simulink model "onlympc"  (R2025a)
settings: Solver=FixedStepAuto  StartTime=0.0  StopTime=inf  FixedStep=0.01  RelTol=1e-3  EnableMultiTasking=on
InitFcn:
  | load2slx
model workspace (MAT data in the model file):
  F = [1.0101  0  0; 0  1.0101  0; 0  0  1.0101; 1.02030201  0  0; 0  1.02030201  0; 0  0  1.02030201; 1.0306070603  0  0; 0  1.0306070603  0; 0  0  1.0306070603; 1.04101619161  0  0; 0  1.04101619161  0; 0  0  1.04101619161; 1.05153045515  0  0; 0  1.05153045515  0; 0  0  1.05153045515]
  G = [0.3357  0  0  0  0  0  0  0  0  0  0  0  0  0  0; 0  0.9698  0  0  0  0  0  0  0  0  0  0  0  0  0; 0  0  0.0305  0  0  0  0  0  0  0  0  0  0  0  0; 0.33909057  0  0  0.3357  0  0  0  0  0  0  0  0  0  0  0; 0  0.97959498  0  0  0.9698  0  0  0  0  0  0  0  0  0  0; 0  0  0.03080805  0  0  0.0305  0  0  0  0  0  0  0  0  0; 0.342515384757  0  0  0.33909057  0  0  0.3357  0  0  0  0  0  0  0  0; 0  0.989488889298  0  0  0.97959498  0  0  0.9698  0  0  0  0  0  0  0; 0  0  0.031119211305  0  0  0.03080805  0  0  0.0305  0  0  0  0  0  0; 0.345974790143  0  0  0.342515384757  0  0  0.33909057  0  0  0.3357  0  0  0  0  0; 0  0.99948272708  0  0  0.989488889298  0  0  0.97959498  0  0  0.9698  0  0  0  0; 0  0  0.0314335153392  0  0  0.031119211305  0  0  0.03080805  0  0  0.0305  0  0  0; 0.349469135523  0  0  0.345974790143  0  0  0.342515384757  0  0  0.33909057  0  0  0.3357  0  0; 0  1.00957750262  0  0  0.99948272708  0  0  0.989488889298  0  0  0.97959498  0  0  0.9698  0; 0  0  0.0317509938441  0  0  0.0314335153392  0  0  0.031119211305  0  0  0.03080805  0  0  0.0305]
  H = [4.19586686919 -9.80424066465e-17 0 1.07234172774 -9.70620796422e-17 0 0.948924882083 -9.60915549373e-17 0 0.82560386835 -9.51307345186e-17 0 ... (225 elements, 15x15)]
  Pc = [-0.3357 0 0 0.3357 0 0 -0.33909057 0 0 0.33909057 0 0 ... (990 elements, 66x15)]
  Qvec = [1  0  0  0  0  0  0  0  0  0  0  0  0  0  0; 0  1  0  0  0  0  0  0  0  0  0  0  0  0  0; 0  0  1  0  0  0  0  0  0  0  0  0  0  0  0; 0  0  0  1  0  0  0  0  0  0  0  0  0  0  0; 0  0  0  0  1  0  0  0  0  0  0  0  0  0  0; 0  0  0  0  0  1  0  0  0  0  0  0  0  0  0; 0  0  0  0  0  0  1  0  0  0  0  0  0  0  0; 0  0  0  0  0  0  0  1  0  0  0  0  0  0  0; 0  0  0  0  0  0  0  0  1  0  0  0  0  0  0; 0  0  0  0  0  0  0  0  0  1  0  0  0  0  0; 0  0  0  0  0  0  0  0  0  0  1  0  0  0  0; 0  0  0  0  0  0  0  0  0  0  0  1  0  0  0; 0  0  0  0  0  0  0  0  0  0  0  0  5.98692002709  -2.77885236035e-16  0; 0  0  0  0  0  0  0  0  0  0  0  0  -2.77885236035e-16  2.39602599551  0; 0  0  0  0  0  0  0  0  0  0  0  0  0  0  99.0360453232]
  Sc = [1.0101  0  0; 0  1.0101  0; 0  0  1.0101; -1.0101  0  0; 0  -1.0101  0; 0  0  -1.0101; 1.02030201  0  0; 0  1.02030201  0; 0  0  1.02030201; -1.02030201  0  0; 0  -1.02030201  0; 0  0  -1.02030201; 1.0306070603  0  0; 0  1.0306070603  0; 0  0  1.0306070603; -1.0306070603  0  0; 0  -1.0306070603  0; 0  0  -1.0306070603; 1.04101619161  0  0; 0  1.04101619161  0; 0  0  1.04101619161; -1.04101619161  0  0; 0  -1.04101619161  0; 0  0  -1.04101619161; 1.05153045515  0  0; 0  1.05153045515  0; 0  0  1.05153045515; -1.05153045515  0  0; 0  -1.05153045515  0; 0  0  -1.05153045515; 0  0  0; 0  0  0; 0  0  0; 0  0  0; 0  0  0; 0  0  0; 0  0  0; 0  0  0; 0  0  0; 0  0  0; 0  0  0; 0  0  0; 0  0  0; 0  0  0; 0  0  0; 0  0  0; 0  0  0; 0  0  0; 0  0  0; 0  0  0; 0  0  0; 0  0  0; 0  0  0; 0  0  0; 0  0  0; 0  0  0; 0  0  0; 0  0  0; 0  0  0; 0  0  0; 1.05153045515  0  0; 0  1.05153045515  0; 0  0  1.05153045515; -1.05153045515  0  0; 0  -1.05153045515  0; 0  0  -1.05153045515]
  m = 3
  nu = 15
  qc = [1; 1; 1; 1; 1; 1; 1; 1; 1; 1; 1; 1; 1; 1; 1; 1; 1; 1; 1; 1; 1; 1; 1; 1; 1; 1; 1; 1; 1; 1; 1.41421356237; 1.41421356237; 2; 1.41421356237; 1.41421356237; 2; 1.41421356237; 1.41421356237; 2; 1.41421356237; 1.41421356237; 2; 1.41421356237; 1.41421356237; 2; 1.41421356237; 1.41421356237; 2; 1.41421356237; 1.41421356237; 2; 1.41421356237; 1.41421356237; 2; 1.41421356237; 1.41421356237; 2; 1.41421356237; 1.41421356237; 2; 1; 1; 1; 1; 1; 1]
undefined symbols (not defined in the file or in its folder): dspblkCoreblockFVToolHelper, gcbh
libraries: px4Peripheralslib x1, px4Sensorslib x1
settings Model: SimulationMode=external  ExtModeTrigDuration=10  Creator=The MathWorks, Inc.  LastModifiedBy=aero
settings SolverCC: AlgebraicLoopSolver=TrustRegion  PositivePriorityOrder=on  AutoInsertRateTranBlk=on  MaxZcPerStep=1.0
settings OptimizationCC: EnhancedBackFolding=on  PassReuseOutputArgsAs=Individual arguments  MaxStackSize=64  OptimizeBlockOrder=speed  DifferentSizesBufferReuse=on  OptimizationCustomize=off  EfficientTunableParamExpr=on
settings DebuggingCC: ParameterPrecisionLossMsg=none  ParameterTunabilityLossMsg=error  UnconnectedInputMsg=warning  UnconnectedOutputMsg=warning  UnconnectedLineMsg=warning  SubsystemReferenceDiagnosticForUnitTest=warning  ArithmeticOperatorsInVariantConditions=warning
settings HardwareCC: ProdBitPerPointer=32.0  ProdBitPerSizeT=32.0  ProdBitPerPtrDiffT=32.0  ProdLargestAtomicInteger=Long  ProdLargestAtomicFloat=Double  ProdWordSize=32.0  ProdLongLongMode=on  ProdHWDeviceType=ARM Compatible->ARM Cortex
settings ModelReferenceCC: EnableRefExpFcnMdlSchedulingChecks=on
settings SFSimCC: MATLABDynamicMemAlloc=off  SimTargetLang=C++  SimDLTargetLibrary=mkl-dnn
settings RTWCC: SystemTargetFile=ert.tlc  HardwareBoard=PX4 Pixhawk 6c  TLCOptions="-aInlineSetEventsForThisBaseRateFcn=TLC_FALSE -aSuppressMultiTaskScheduler=TLC_FALSE  -aRateBasedStepFcn=0"  TemplateMakefile=ert_default_tmf  GenerateReport=on  Toolchain=GNU Tools for PX4 Autopilots  BuildConfiguration=Faster Runs  IncludeHyperlinkInReport=on  LaunchReport=on  TargetLang=C++  GenerateTraceInfo=on  GenerateTraceReport=on  GenerateTraceReportSl=on  GenerateTraceReportSf=on  GenerateTraceReportEml=on  GPUComputeCapability=3.5  DLArmComputeVersion=19.05  Description=Embedded Coder
settings CodeAppCC: ForceParamTrailComments=on  IgnoreCustomStorageClasses=off  OperatorAnnotations=on  SimulinkDataObjDesc=on  SFDataObjDesc=on  InsertBlockDesc=on
settings ERTTargetCC: ExtModeTransport=3.0  ExtModeStaticAllocSize=1024.0  InlinedParameterPlacement=Hierarchical

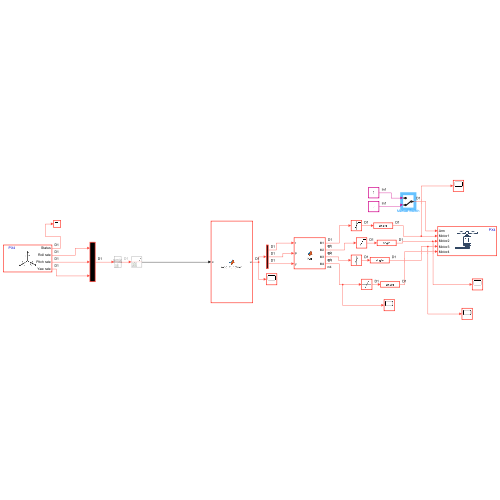
[thumbnail: Simulink's stored preview of the top-level diagram]
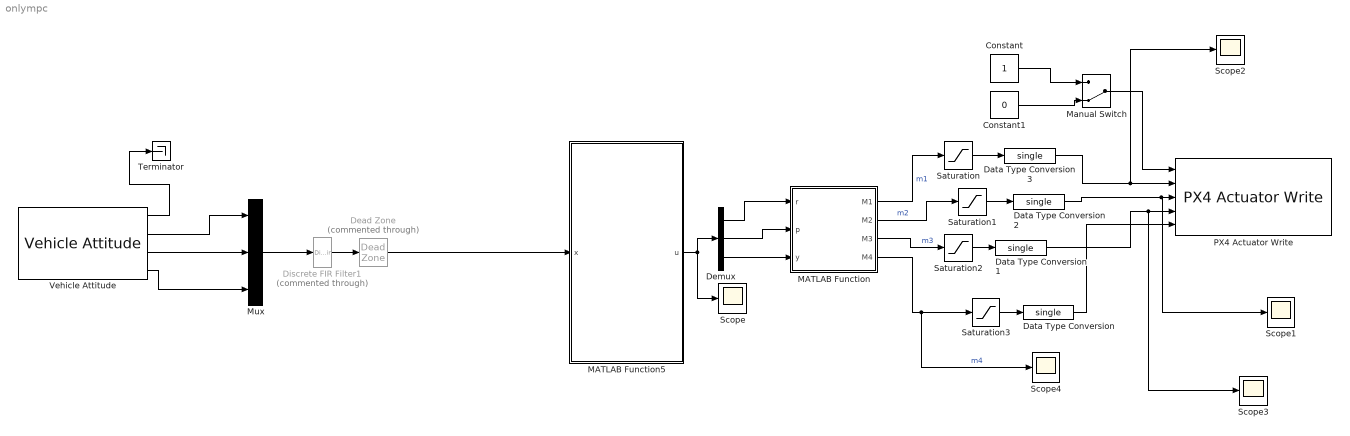
== system onlympc ==
  Constant : Constant  OutDataTypeStr=boolean
  Constant1 : Constant  Value=0  OutDataTypeStr=boolean
  Data Type Conversion{,1..3} (4 alike) : DataTypeConversion  OutDataTypeStr=single  SaturateOnIntegerOverflow=off  RndMeth=Floor
  Dead Zone : DeadZone  Commented=through  LowerValue=-0.017  UpperValue=0.017
  Demux : Demux  Outputs=3
  Discrete FIR Filter1 : DiscreteFir  Commented=through  LoadFcn=dspblkCoreblockFVToolHelper(gcbh,'load');  Coefficients=[0.2 0.2 0.2 0.2 0.2]
      settings: CopyFcn=dspblkCoreblockFVToolHelper(gcbh,'copy');  DeleteFcn=dspblkCoreblockFVToolHelper(gcbh,'close');  ModelCloseFcn=dspblkCoreblockFVToolHelper(gcbh,'close');  PreSaveFcn=dspblkCoreblockFVToolHelper(gcbh,'presave');  PostSaveFcn=dspblkCoreblockFVToolHelper(gcbh,'postsave');  CloseFcn=dspblkCoreblockFVToolHelper(gcbh,'close');
  MATLAB Function : MATLAB Function  TreatAsAtomicUnit=on
  MATLAB Function5 : MATLAB Function  TreatAsAtomicUnit=on  SystemSampleTime=0.01
  Manual Switch : ManualSwitch  CurrentSetting=0
  Mux : Mux  Inputs=3
  PX4 Actuator Write : px4Peripheralslib/PX4 Actuator Write  Motor1Enable=on  Motor2Enable=on  Motor3Enable=on  Motor4Enable=on  Motor5Enable=off  Motor6Enable=off  Motor7Enable=off  Motor8Enable=off  Motor9Enable=off  Motor10Enable=off  Motor11Enable=off  Motor12Enable=off  IsMotorArray=off  Servo1Enable=off  Servo2Enable=off  Servo3Enable=off  Servo4Enable=off  Servo5Enable=off  Servo6Enable=off  Servo7Enable=off  Servo8Enable=off  IsServoArray=off
  Saturation{,1..3} (4 alike) : Saturate  UpperLimit=1  LowerLimit=0
  Scope{,1..4} (5 alike) : Scope
      Scope settings: ActiveDisplayYMinimum=-0.20094468799626919  ActiveDisplayYMaximum=0.25880684258194991
      Scope1 settings: ActiveDisplayYMinimum=0.204619275406003  ActiveDisplayYMaximum=0.21324986033141613
      Scope2 settings: ActiveDisplayYMinimum=0.00829335488379003  ActiveDisplayYMaximum=0.64960764907300472  DataLoggingVariableName=ScopeData2
      Scope3 settings: ActiveDisplayYMinimum=0.086084697037949576  ActiveDisplayYMaximum=0.57265901246140893  DataLoggingVariableName=ScopeData3
      Scope4 settings: ActiveDisplayYMinimum=0.09643536073618425  ActiveDisplayYMaximum=0.86308686784221988  DataLoggingVariableName=ScopeData4
  Terminator : Terminator
  Vehicle Attitude : px4Sensorslib/Vehicle Attitude  rollRate=on  pitchRate=on  yawRate=on  quaternion=off  uorbTimeStamp=off  BlockingMode=off  BlockTimeout=0.001  sampleTime=0.01
  wires:
  MATLAB Function/2(M2) -> Saturation1/1  "m2"
  Demux/3 -> MATLAB Function/3(y)
  Demux/1 -> MATLAB Function/1(r)
  MATLAB Function5/1(u) -> Demux/1, Scope/1
  MATLAB Function/1(M1) -> Saturation/1  "m1"
  MATLAB Function/4(M4) -> Scope4/1, Saturation3/1  "m4"
  Demux/2 -> MATLAB Function/2(p)
  MATLAB Function/3(M3) -> Saturation2/1  "m3"
  Vehicle Attitude/1 -> Terminator/1
  Vehicle Attitude/2 -> Mux/1
  Vehicle Attitude/3 -> Mux/2
  Vehicle Attitude/4 -> Mux/3
  Saturation/1 -> Data Type Conversion3/1
  Saturation1/1 -> Data Type Conversion2/1
  Saturation2/1 -> Data Type Conversion1/1
  Saturation3/1 -> Data Type Conversion/1
  Discrete FIR Filter1/1 -> Dead Zone/1
  Mux/1 -> Discrete FIR Filter1/1
  Dead Zone/1 -> MATLAB Function5/1(x)
  Data Type Conversion/1 -> PX4 Actuator Write/5
  Data Type Conversion1/1 -> Scope3/1, PX4 Actuator Write/4
  Data Type Conversion2/1 -> Scope1/1, PX4 Actuator Write/3
  Data Type Conversion3/1 -> Scope2/1, PX4 Actuator Write/2
  Constant1/1 -> Manual Switch/2
  Constant/1 -> Manual Switch/1
  Manual Switch/1 -> PX4 Actuator Write/1

== matlab function onlympc/MATLAB Function ==
  data: M1 output; r input; p input; y input; M2 output; M3 output; M4 output
function [M1,M2,M3,M4] = fcn( r, p, y)
% t: thrust
% r: roll
% p: pitch
% y: yaw
persistent trim mixer thrust
% M1 = t + r + p - y;
% M2 = t - r - p - y;
% M3 = t - r + p + y;
% M4 = t + r - p + y;
trim = [0.1344;0.2078;0.1551;0.2548];
thrust = 0;
u = [r;p;y; thrust];
mixer = [-1 1 1 -1;
        1 -1 1 -1;
        1 1 -1 -1
        1 1 1 1];
M = mixer\u;
M1= M(1,1)+trim(1,1);
M2= M(2,1)+trim(2,1);
M3= M(3,1)+trim(3,1);
M4= M(4,1)+trim(4,1);

== matlab function onlympc/MATLAB Function5 ==
  data: x input; u output size=[m 1]; H parameter double; F parameter double; Qvec parameter double; G parameter double; Pc parameter double; qc parameter double; Sc parameter double
function u = mpc_function(x, H, F, Qvec, G, Pc, qc, Sc)
persistent opts x0 u_prev
x = double(x);
if isempty(u_prev)
    u_prev = zeros(3,1,'double');
end

if isempty(x0)
    x0 = zeros(15,1,'double');
end
% uvec = zeros(nu,1);

% === Construcción del QP ===
f = (2*x'*F'*Qvec*G)';

% Resolver QP
if isempty(opts)
opts = optimoptions('quadprog', 'Algorithm','active-set','Display','off');
end
[uvec,a,b] = quadprog(2*H,f, Pc,qc + Sc*x,[],[],[],[],x0, opts);

% Acción de control 
u = zeros(3,1);
if  b > 0
uvec = double(uvec);
u(:) = uvec(1:3);
u_prev = u;
x0= uvec;
else
    u = u_prev;
end
